simulink model "steeringSimulationSimplified"  (R2015b)
settings: Solver=ode45  StartTime=0.0  StopTime=20  RelTol=1e-3
libraries: simulink x1
settings Model: Creator=vniel  LastModifiedBy=Thomas
settings DataIOCC: SaveFormat=Array
settings HardwareCC: ProdBitPerPointer=32  ProdLargestAtomicFloat=None  ProdIntDivRoundTo=Undefined  ProdEndianess=Unspecified  ProdWordSize=32  ProdHWDeviceType=32-bit Generic
settings GRTTargetCC: GeneratePreprocessorConditionals=Disable all
settings ConfigComp: CovModelRefEnable=Off

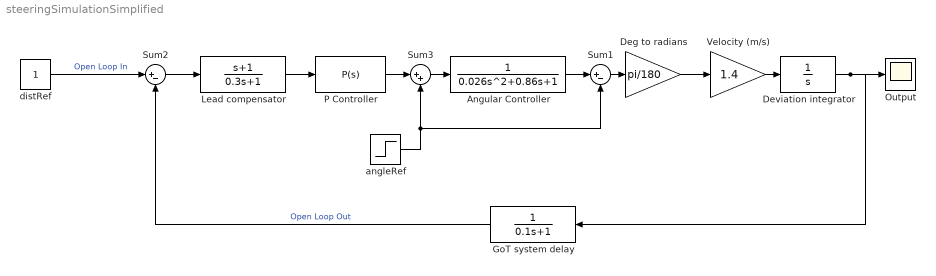
== system steeringSimulationSimplified ==
  Angular Controller : TransferFcn  Denominator=[0.026 0.86 1]
  Deg to radians : Gain  Gain=pi/180
  Deviation integrator : TransferFcn  Denominator=[1 0]
  GoT system delay : TransferFcn  Denominator=[0.1 1]
  Lead compensator : TransferFcn  Numerator=[1 1]  Denominator=[0.3 1]
  Output : Scope
  P Controller : simulink/Continuous/PID Controller  Controller=P  TimeDomain=Continuous-time  SampleTime=-1  IntegratorMethod=Forward Euler  FilterMethod=Forward Euler  Form=Parallel  UseFilter=on  ControllerParametersSource=internal  P=48.87  I=0  D=0  N=0  InitialConditionSource=internal  InitialConditionForIntegrator=0  InitialConditionForFilter=0  ExternalReset=none  LimitOutput=on  UpperSaturationLimit=90  LowerSaturationLimit=-90  LinearizeAsGain=on  AntiWindupMode=none  Kb=1  TrackingMode=off  Kt=1  PParamMin=[]  PParamMax=[]  IParamMin=[]  IParamMax=[]  DParamMin=[]  DParamMax=[]  NParamMin=[]  NParamMax=[]  KbParamMin=[]  KbParamMax=[]  KtParamMin=[]  KtParamMax=[]  POutMin=[]  POutMax=[]  IOutMin=[]  IOutMax=[]  DOutMin=[]  DOutMax=[]  NOutMin=[]  NOutMax=[]  KbOutMin=[]  KbOutMax=[]  KtOutMin=[]  KtOutMax=[]  IntegratorOutMin=[]  IntegratorOutMax=[]  FilterOutMin=[]  FilterOutMax=[]  SumOutMin=[]  SumOutMax=[]  SumI1OutMin=[]  SumI1OutMax=[]  SumI2OutMin=[]  SumI2OutMax=[]  SumI3OutMin=[]  SumI3OutMax=[]  SumDOutMin=[]  SumDOutMax=[]  SaturationOutMin=[]  SaturationOutMax=[]  IntegratorContinuousStateAttributes=''  IntegratorStateMustResolveToSignalObject=off  IntegratorRTWStateStorageClass=Auto  FilterContinuousStateAttributes=''  FilterStateMustResolveToSignalObject=off  FilterRTWStateStorageClass=Auto  DifferentiatorICPrevScaledInput=0  DifferentiatorOutMin=[]  DifferentiatorOutMax=[]
  Sum1 : Sum  Inputs=|+-
  Sum2 : Sum  Inputs=|+-
  Sum3 : Sum  Inputs=|++
  Velocity (m/s) : Gain  Gain=1.4
  angleRef : Step  Time=5  After=0  SampleTime=0
  distRef : Constant
  wires:
  angleRef/1 -> Sum1/2, Sum3/2
  distRef/1 -> Sum2/1  "Open Loop In"
  Velocity (m/s)/1 -> Deviation integrator/1
  Sum1/1 -> Deg to radians/1
  P Controller/1 -> Sum3/1
  Deviation integrator/1 -> GoT system delay/1, Output/1
  GoT system delay/1 -> Sum2/2  "Open Loop Out"
  Sum3/1 -> Angular Controller/1
  Angular Controller/1 -> Sum1/1
  Sum2/1 -> Lead compensator/1
  Deg to radians/1 -> Velocity (m/s)/1
  Lead compensator/1 -> P Controller/1
